simulink model "lvservomtr_dq_plant"  (R2025b)
settings: Solver=VariableStepAuto  StartTime=0.0  StopTime=0.08  RelTol=1e-3
undefined symbols (not defined in the file): motor
settings Model: Creator=semih  LastModifiedBy=semih

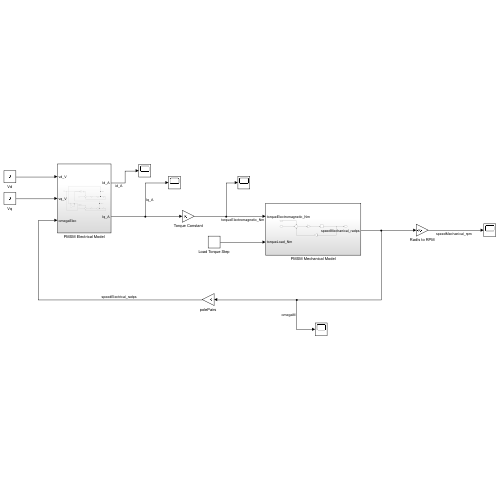
[thumbnail: Simulink's stored preview of the top-level diagram]
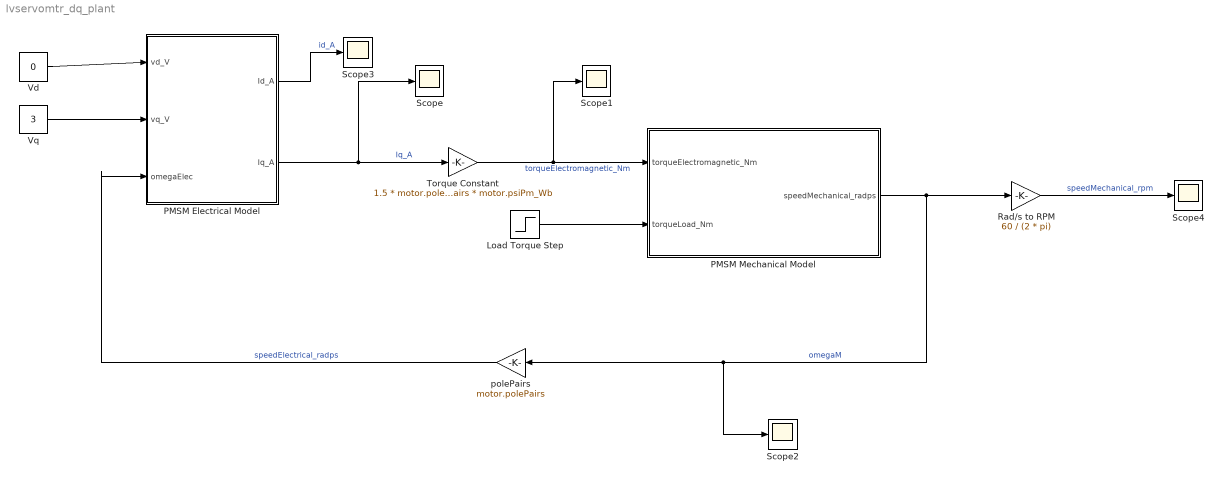
== system lvservomtr_dq_plant ==
  Load Torque Step : Step  Time=0.030  After=0.05  SampleTime=0
  PMSM Electrical Model : Subsystem
  PMSM Mechanical Model : Subsystem
  Rad/s to RPM : Gain  Gain=60 / (2 * pi)
  Scope{,1..4} (5 alike) : Scope
      Scope settings: ActiveDisplayYMinimum=-0.42366511792142403  ActiveDisplayYMaximum=1.8876545573518515
      Scope1 settings: ActiveDisplayYMinimum=-1  ActiveDisplayYMaximum=1
      Scope2 settings: ActiveDisplayYMinimum=-14.648422716149396  ActiveDisplayYMaximum=131.83580444534459  DataLoggingVariableName=ScopeData2
      Scope3 settings: ActiveDisplayYMinimum=-0.077109095292808  ActiveDisplayYMaximum=0.69398185763527209  DataLoggingVariableName=ScopeData3
      Scope4 settings: ActiveDisplayYMinimum=-139.88213302648705  ActiveDisplayYMaximum=1258.9391972383837  DataLoggingVariableName=ScopeData4
  Torque Constant : Gain  Gain=1.5 * motor.polePairs * motor.psiPm_Wb
  Vd : Constant  Value=0
  Vq : Constant  Value=3
  polePairs : Gain  Gain=motor.polePairs
  wires:
  PMSM Electrical Model/2(Iq_A) -> Scope/1, Torque Constant/1  "Iq_A"
  Torque Constant/1 -> Scope1/1, PMSM Mechanical Model/1(torqueElectromagnetic_Nm)  "torqueElectromagnetic_Nm"
  PMSM Mechanical Model/1(speedMechanical_radps) -> Rad/s to RPM/1, Scope2/1, polePairs/1  "omegaM"
  polePairs/1 -> PMSM Electrical Model/3(omegaElec)  "speedElectrical_radps"
  Load Torque Step/1 -> PMSM Mechanical Model/2(torqueLoad_Nm)
  Vd/1 -> PMSM Electrical Model/1(vd_V)
  Vq/1 -> PMSM Electrical Model/2(vq_V)
  PMSM Electrical Model/1(Id_A) -> Scope3/1  "id_A"
  Rad/s to RPM/1 -> Scope4/1  "speedMechanical_rpm"

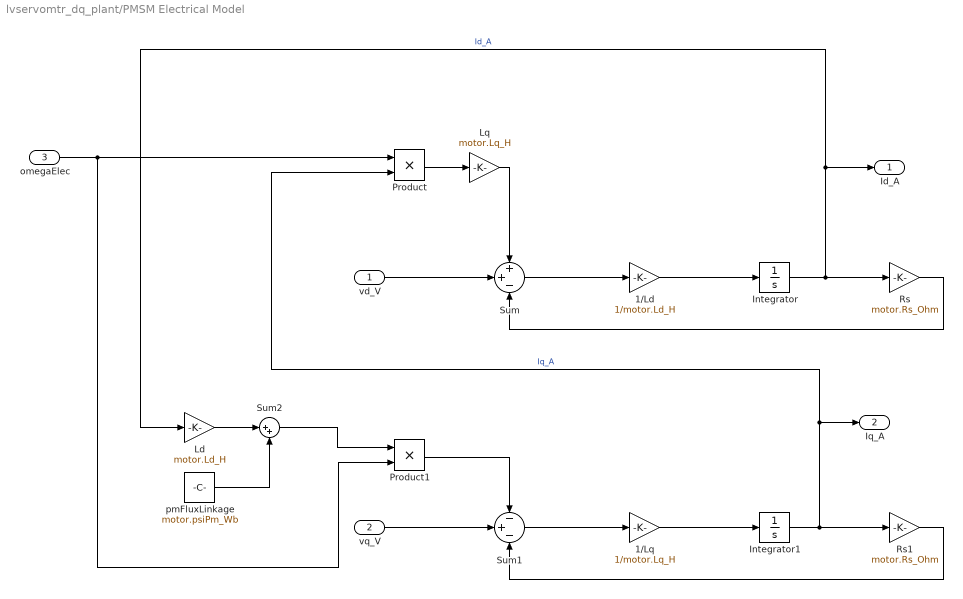
== system lvservomtr_dq_plant/PMSM Electrical Model ==
  vd_V : Inport
  vq_V : Inport  Port=2
  omegaElec : Inport  Port=3
  1/Ld : Gain  Gain=1/motor.Ld_H
  1/Lq : Gain  Gain=1/motor.Lq_H
  Integrator : Integrator  InitialCondition=motor.id0_A
  Integrator1 : Integrator  InitialCondition=motor.iq0_A
  Ld : Gain  Gain=motor.Ld_H
  Lq : Gain  Gain=motor.Lq_H
  Product : Product
  Product1 : Product
  Rs : Gain  Gain=motor.Rs_Ohm
  Rs1 : Gain  Gain=motor.Rs_Ohm
  Sum : Sum  Inputs=++-
  Sum1 : Sum  Inputs=-+-
  Sum2 : Sum  Inputs=|++
  pmFluxLinkage : Constant  Value=motor.psiPm_Wb
  Id_A : Outport
  Iq_A : Outport  Port=2
  wires:
  1/Ld/1 -> Integrator/1
  Integrator1/1 -> Product/2, Iq_A/1, Rs1/1  "Iq_A"
  Sum/1 -> 1/Ld/1
  Rs/1 -> Sum/3
  vq_V/1 -> Sum1/2
  Integrator/1 -> Id_A/1, Ld/1, Rs/1  "Id_A"
  Sum1/1 -> 1/Lq/1
  Product/1 -> Lq/1
  Lq/1 -> Sum/1
  1/Lq/1 -> Integrator1/1
  Rs1/1 -> Sum1/3
  Product1/1 -> Sum1/1
  vd_V/1 -> Sum/2
  Ld/1 -> Sum2/1
  pmFluxLinkage/1 -> Sum2/2
  Sum2/1 -> Product1/1
  omegaElec/1 -> Product1/2, Product/1

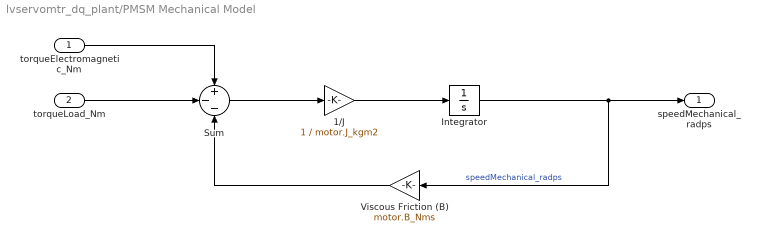
== system lvservomtr_dq_plant/PMSM Mechanical Model ==
  torqueElectromagnetic_Nm : Inport
  torqueLoad_Nm : Inport  Port=2
  1/J : Gain  Gain=1 / motor.J_kgm2
  Integrator : Integrator  InitialCondition=motor.speed0_radps
  Sum : Sum  Inputs=+--
  Viscous Friction (B) : Gain  Gain=motor.B_Nms
  speedMechanical_radps : Outport
  wires:
  torqueElectromagnetic_Nm/1 -> Sum/1
  torqueLoad_Nm/1 -> Sum/2
  Sum/1 -> 1/J/1
  Integrator/1 -> Viscous Friction (B)/1, speedMechanical_radps/1  "speedMechanical_radps"
  1/J/1 -> Integrator/1
  Viscous Friction (B)/1 -> Sum/3
